simulink model "demo1"  (Simulink 3.00)
settings: Solver=ode45  StartTime=0.0  StopTime=10.0  RelTol=1e-3
values from neighbouring files (symbols this model uses):
  p560 =     [matlab.mat]
libraries: simulink3 x1
settings Model: Creator=pic  LastModifiedBy=pic

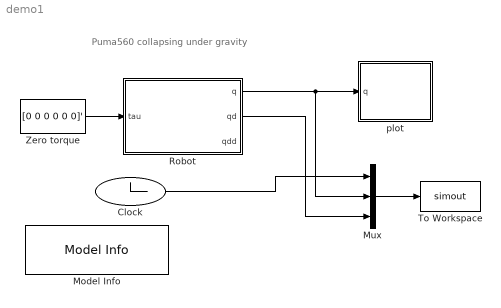
== system demo1 ==
  note: Puma560 collapsing under gravity
  Clock : Clock
      settings: Decimation=10
  Model Info : simulink3/Signals & Systems/Model Info  InitialBlockCM=none  BlockCM=none  Frame=on  DisplayStringWithTags=|  HorizontalTextAlignment=Left  LeftAlignmentValue=0.02  SourceBlockDiagram=demo1  TagMaxNumber=20
      | Simple dynamics demo
      | %<Creator>
      | %<LastModificationDate>
  Mux : Mux  Inputs=3
  Robot : Subsystem  mask{robot=p560, q0=[0 0 0 0 0 0]}
      mask prompts: robot "Robot object"; q0 "Initial state"
      mask help: Dynamic model of robot
      mask init:
      | n = robot.n;
      mask Help: gravity comes from the robot object
      mask Display:
      | text(0.5, 0.8, robot.name, 'horizontalAlignment', 'center')
      | port_label('input', 1, 'tau')
      | port_label('output', 1, 'q')
      | port_label('output', 2, 'qd')
      | port_label('output', 3, 'qdd')
  To Workspace : ToWorkspace  VariableName=simout  SampleTime=-1  SaveFormat=Matrix
  Zero torque : Constant  Value=[0 0 0 0 0 0]'
  plot : Subsystem  mask{robot=p560}
      mask prompts: robot "Name of robot"
      mask init:
      | plot(robot,zeros(1,robot.n))
      mask Help: This block graphically displays the named robot
      mask Display: text(0.5, 0.5,  robot.name, 'horizontalAlignment', 'center')
  wires:
  Zero torque/1 -> Robot/1(tau)
  Mux/1 -> To Workspace/1
  Robot/1(q) -> plot/1(q), Mux/2
  Clock/1 -> Mux/1
  Robot/2(qd) -> Mux/3

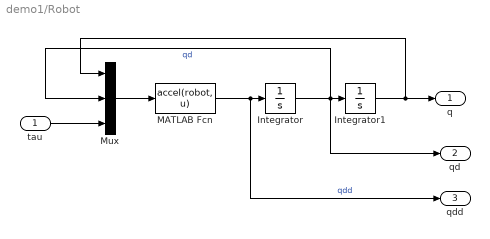
== system demo1/Robot ==
  tau : Inport  Port=1  PortWidth=-1  SampleTime=-1  DataType=auto
      settings: SignalType=auto
  Integrator : Integrator  ExternalReset=none  InitialConditionSource=internal  InitialCondition=0  LimitOutput=off  UpperSaturationLimit=inf  LowerSaturationLimit=-inf  ShowSaturationPort=off  ShowStatePort=off  AbsoluteTolerance=auto
  Integrator1 : Integrator  ExternalReset=none  InitialConditionSource=internal  InitialCondition=0  LimitOutput=off  UpperSaturationLimit=inf  LowerSaturationLimit=-inf  ShowSaturationPort=off  ShowStatePort=off  AbsoluteTolerance=auto
  MATLAB Fcn : MATLABFcn  MATLABFcn=accel(robot, u)  OutputWidth=n  OutputSignalType=real
  Mux : Mux  Inputs=3
  q : Outport  Port=1
  qd : Outport  Port=2
  qdd : Outport  Port=3
  wires:
  MATLAB Fcn/1 -> qdd/1, Integrator/1  "qdd"
  Mux/1 -> MATLAB Fcn/1
  Integrator/1 -> qd/1, Integrator1/1, Mux/2  "qd"
  tau/1 -> Mux/3
  Integrator1/1 -> q/1, Mux/1

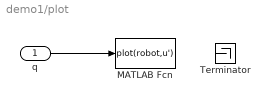
== system demo1/plot ==
  q : Inport  Port=1  PortWidth=-1  SampleTime=-1  DataType=auto
      settings: SignalType=auto
  MATLAB Fcn : MATLABFcn  MATLABFcn=plot(robot,u')  OutputWidth=0  OutputSignalType=auto
  Terminator : Terminator
  wires:
  ? -> Terminator/1
  q/1 -> MATLAB Fcn/1
